simulink model "model_cessna182_ld"  (R2013a)
settings: Solver=ode45  StartTime=0.0  StopTime=100  MaxStep=0.01  RelTol=1e-3
InitFcn:
  | cessna182
values from neighbouring files (symbols this model uses):
  Cld = eye(4)    [cessna182.m]
  Dld = zeros (4,2)    [cessna182.m]
  Kp = 12    [cessna182_ld.m]
  Kr = 10    [cessna182_ld.m]
undefined symbols (not defined in the file or in its folder): Ald, Bld
settings Model: Creator=Aluno  LastModifiedBy=Aluno

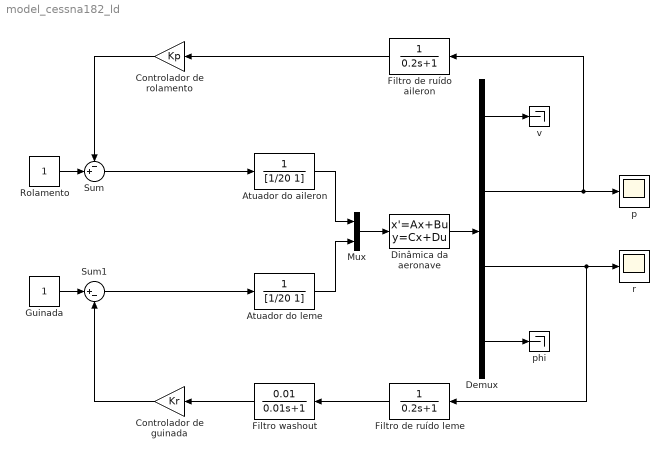
== system model_cessna182_ld ==
  Atuador do aileron : TransferFcn  Denominator=[1/20 1]
  Atuador do leme : TransferFcn  Denominator=[1/20 1]
  Controlador de guinada : Gain  Gain=Kr
  Controlador de rolamento : Gain  Gain=Kp
  Demux : Demux
  Dinâmica da aeronave : StateSpace  A=Ald  B=Bld  C=Cld  D=Dld
  Filtro de ruído aileron : TransferFcn  Denominator=[0.2 1]
  Filtro de ruído leme : TransferFcn  Denominator=[0.2 1]
  Filtro washout : TransferFcn  Numerator=[0.01]  Denominator=[0.01 1]
  Guinada : Constant
  Mux : Mux  Inputs=2
  Rolamento : Constant
  Sum : Sum  Inputs=-+|
  Sum1 : Sum  Inputs=|+-
  p : Scope
      settings: YMin=-0.25  YMax=4.5  SaveName=p
  phi : Terminator
  r : Scope
      settings: SaveName=r
  v : Terminator
  wires:
  Mux/1 -> Dinâmica da aeronave/1
  Dinâmica da aeronave/1 -> Demux/1
  Demux/1 -> v/1
  Demux/4 -> phi/1
  Demux/2 -> p/1, Filtro de ruído aileron/1
  Demux/3 -> r/1, Filtro de ruído leme/1
  Atuador do aileron/1 -> Mux/1
  Atuador do leme/1 -> Mux/2
  Filtro de ruído aileron/1 -> Controlador de rolamento/1
  Controlador de rolamento/1 -> Sum/1
  Rolamento/1 -> Sum/2
  Sum/1 -> Atuador do aileron/1
  Guinada/1 -> Sum1/1
  Sum1/1 -> Atuador do leme/1
  Controlador de guinada/1 -> Sum1/2
  Filtro de ruído leme/1 -> Filtro washout/1
  Filtro washout/1 -> Controlador de guinada/1
